simulink model "CruiseControlWebsite"  (Simulink 8.7)
settings: Solver=ode45  StartTime=0.0  StopTime=100  MaxStep=0.1  RelTol=1e-3
PreLoadFcn:
  | m = 1000;
  | alpha = [40, 25, 16, 12, 10];
  | Tm = 190;
  | wm = 420;
  | beta = 0.4;
  | Cr = 0.01;
  | rho = 1.3;
  | Cd = 0.32;
  | A = 2.4;
  | g = 9.8;
  | theta = 0;
  | gear = 3;
libraries: simulink x1
settings Model: Creator=Cole Lepine  LastModifiedBy=Juan Antonio  ExtModeAutoUpdateStatusClock=off
settings DataIOCC: SignalLoggingSaveFormat=ModelDataLogs
settings OptimizationCC: ExpressionDepthLimit=2147483647  InitFltsAndDblsToZero=on
settings DebuggingCC: SaveWithParameterizedLinksMsg=none  SolverPrmCheckMsg=warning  FcnCallInpInsideContextMsg=UseLocalSettings  StateNameClashWarn=warning
settings GRTTargetCC: GeneratePreprocessorConditionals=Use local settings  CombineOutputUpdateFcns=off  GRTInterface=on

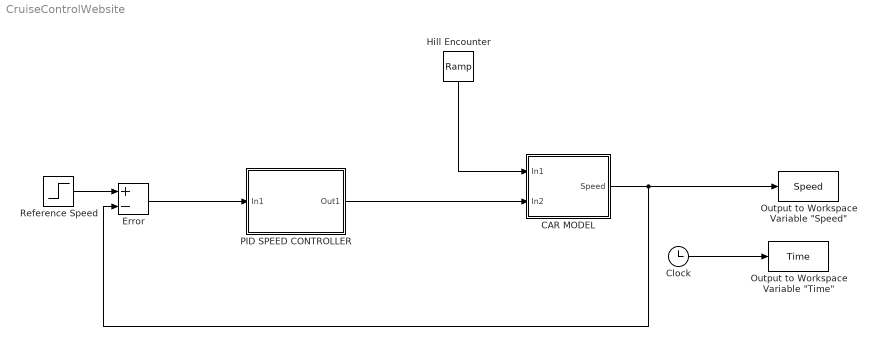
== system CruiseControlWebsite ==
  CAR MODEL : Subsystem
  Clock : Clock
  Error : Sum  Inputs=+-
  Hill Encounter : simulink/Sources/Ramp  slope=0  start=0  X0=0
  "Output to Workspace Variable \"Time\"" : ToWorkspace  VariableName=Time  SampleTime=-1
  "Output to Workspace Variable \"Speed\"" : ToWorkspace  VariableName=Speed  SampleTime=-1
  PID SPEED CONTROLLER : Subsystem
  Reference Speed : Step  Time=0  Before=40  After=50  SampleTime=0
  wires:
  Reference Speed/1 -> Error/1
  PID SPEED CONTROLLER/1(Out1) -> CAR MODEL/2(In2)
  Clock/1 -> "Output to Workspace Variable \"Time\""/1
  Hill Encounter/1 -> CAR MODEL/1(In1)
  CAR MODEL/1(Speed) -> "Output to Workspace Variable \"Speed\""/1, Error/2
  Error/1 -> PID SPEED CONTROLLER/1(In1)

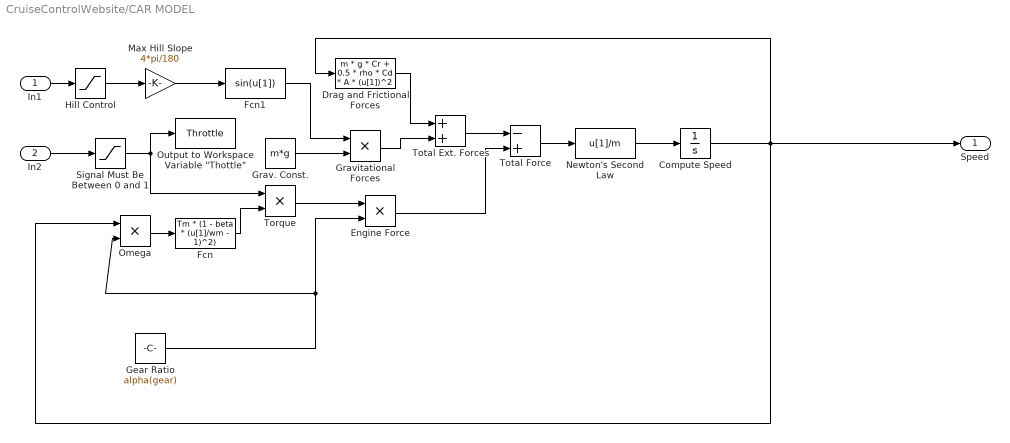
== system CruiseControlWebsite/CAR MODEL ==
  In1 : Inport
  In2 : Inport  Port=2
  Compute Speed : Integrator  InitialCondition=40  ZeroCross=off
  Drag and Frictional Forces : Fcn  Expr=m * g * Cr + 0.5 * rho * Cd * A * (u[1])^2
  Engine Force : Product  Inputs=**
  Fcn : Fcn  Expr=Tm * (1 - beta * (u[1]/wm - 1)^2)
  Fcn1 : Fcn
  Gear Ratio : Constant  Value=alpha(gear)
  Grav. Const. : Constant  Value=m*g
  Gravitational Forces : Product  RndMeth=Zero
  Hill Control : Saturate  UpperLimit=1  LowerLimit=0
  Max Hill Slope : Gain  Gain=4*pi/180
  Newton's Second Law : Fcn  Expr=u[1]/m
  Omega : Product  RndMeth=Zero
  "Output to Workspace Variable \"Thottle\"" : ToWorkspace  VariableName=Throttle  SampleTime=-1
  Signal Must Be Between 0 and 1 : Saturate  UpperLimit=1  LowerLimit=0
  Torque : Product  RndMeth=Zero
  Total Ext. Forces : Sum
  Total Force : Sum  Inputs=-+
  Speed : Outport
  wires:
  Engine Force/1 -> Total Force/2
  Total Force/1 -> Newton's Second Law/1
  Newton's Second Law/1 -> Compute Speed/1
  Compute Speed/1 -> Speed/1, Omega/1, Drag and Frictional Forces/1
  Gear Ratio/1 -> Engine Force/2, Omega/2
  Omega/1 -> Fcn/1
  Torque/1 -> Engine Force/1
  Fcn/1 -> Torque/2
  Signal Must Be Between 0 and 1/1 -> Torque/1, "Output to Workspace Variable \"Thottle\""/1
  Total Ext. Forces/1 -> Total Force/1
  Drag and Frictional Forces/1 -> Total Ext. Forces/1
  Gravitational Forces/1 -> Total Ext. Forces/2
  Fcn1/1 -> Gravitational Forces/1
  Max Hill Slope/1 -> Fcn1/1
  Grav. Const./1 -> Gravitational Forces/2
  Hill Control/1 -> Max Hill Slope/1
  In1/1 -> Hill Control/1
  In2/1 -> Signal Must Be Between 0 and 1/1

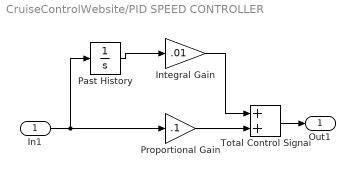
== system CruiseControlWebsite/PID SPEED CONTROLLER ==
  In1 : Inport
  Integral Gain : Gain  Gain=.01
  Past History : Integrator  ZeroCross=off
  Proportional Gain : Gain  Gain=.1
  Total Control Signal : Sum
  Out1 : Outport
  wires:
  Proportional Gain/1 -> Total Control Signal/2
  Integral Gain/1 -> Total Control Signal/1
  In1/1 -> Past History/1, Proportional Gain/1
  Past History/1 -> Integral Gain/1
  Total Control Signal/1 -> Out1/1
